simulink model "psicontrol"  (R2016a)
settings: Solver=VariableStepAuto  StartTime=0.0  StopTime=100  RelTol=1e-3
undefined symbols (not defined in the file): A, B, C, D
settings Model: Creator=Gray  LastModifiedBy=Gray

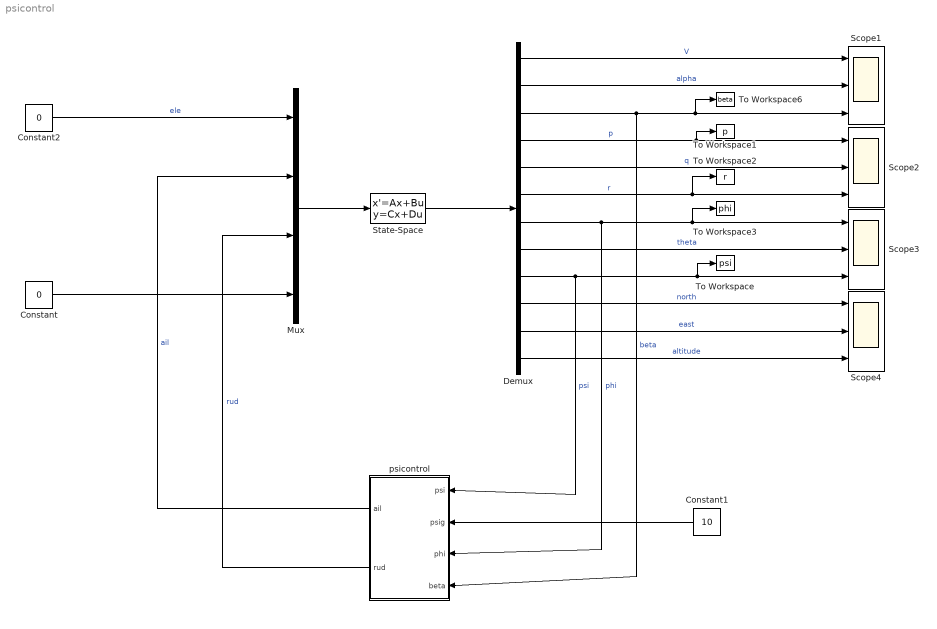
== system psicontrol ==
  Constant : Constant  Value=0
  Constant1 : Constant  Value=10
  Constant2 : Constant  Value=0
  Demux : Demux  Outputs=12
  Mux : Mux
  Scope{1..4} (4 alike) : Scope  NumInputPorts=3
  State-Space : StateSpace  A=A  B=B  C=C  D=D  X0=[0 0 0 0 0 0 0 0 0 0 0 0]
  To Workspace : ToWorkspace  VariableName=psi  SaveFormat=Timeseries  SampleTime=-1
  To Workspace1 : ToWorkspace  VariableName=p  SaveFormat=Timeseries  SampleTime=-1
  To Workspace2 : ToWorkspace  VariableName=r  SaveFormat=Timeseries  SampleTime=-1
  To Workspace3 : ToWorkspace  VariableName=phi  SaveFormat=Timeseries  SampleTime=-1
  To Workspace6 : ToWorkspace  VariableName=beta  SaveFormat=Timeseries  SampleTime=-1
  psicontrol : Subsystem
  wires:
  State-Space/1 -> Demux/1
  Mux/1 -> State-Space/1
  Demux/1 -> Scope1/1  "V"
  Demux/2 -> Scope1/2  "alpha"
  Demux/3 -> psicontrol/4(beta), To Workspace6/1, Scope1/3  "beta"
  Demux/4 -> To Workspace1/1, Scope2/1  "p"
  Demux/5 -> Scope2/2  "q"
  Demux/6 -> To Workspace2/1, Scope2/3  "r"
  Demux/7 -> psicontrol/3(phi), To Workspace3/1, Scope3/1  "phi"
  Demux/8 -> Scope3/2  "theta"
  Demux/9 -> psicontrol/1(psi), To Workspace/1, Scope3/3  "psi"
  Demux/10 -> Scope4/1  "north"
  Demux/11 -> Scope4/2  "east"
  Demux/12 -> Scope4/3  "altitude"
  Constant/1 -> Mux/4
  Constant1/1 -> psicontrol/2(psig)
  Constant2/1 -> Mux/1  "ele"
  psicontrol/2(rud) -> Mux/3  "rud"
  psicontrol/1(ail) -> Mux/2  "ail"

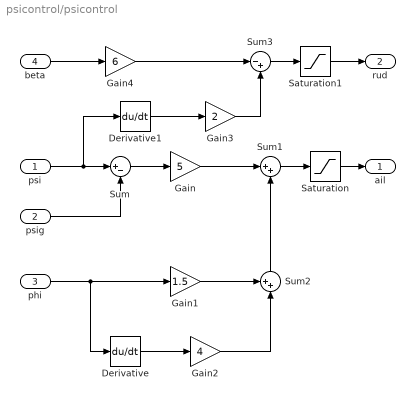
== system psicontrol/psicontrol ==
  psi : Inport
  psig : Inport  Port=2
  phi : Inport  Port=3
  beta : Inport  Port=4
  Derivative : Derivative
  Derivative1 : Derivative
  Gain : Gain  Gain=5
  Gain1 : Gain  Gain=1.5
  Gain2 : Gain  Gain=4
  Gain3 : Gain  Gain=2
  Gain4 : Gain  Gain=6
  Saturation : Saturate  UpperLimit=12  LowerLimit=-12
  Saturation1 : Saturate  UpperLimit=8  LowerLimit=-8
  Sum : Sum  Inputs=|+-
  Sum1 : Sum  Inputs=|++
  Sum2 : Sum  Inputs=++|
  Sum3 : Sum  Inputs=|-+
  ail : Outport
  rud : Outport  Port=2
  wires:
  psig/1 -> Sum/2
  Gain2/1 -> Sum2/2
  Sum2/1 -> Sum1/2
  Derivative1/1 -> Gain3/1
  phi/1 -> Derivative/1, Gain1/1
  Derivative/1 -> Gain2/1
  Gain1/1 -> Sum2/1
  beta/1 -> Gain4/1
  Gain4/1 -> Sum3/1
  Gain3/1 -> Sum3/2
  psi/1 -> Derivative1/1, Sum/1
  Gain/1 -> Sum1/1
  Sum/1 -> Gain/1
  Saturation/1 -> ail/1
  Sum1/1 -> Saturation/1
  Sum3/1 -> Saturation1/1
  Saturation1/1 -> rud/1
